simulink model "UZ_EnDat_be4_adding_bidirectional_clk_shift"  (R2024a)
settings: Solver=FixedStepDiscrete  StartTime=0  StopTime=0.02  FixedStep=1.0E-8  RelTol=1e-3
model workspace (MAT data in the model file):
  Select = 0
libraries: hdlsllib x776, simulink x28, simulink_extras x3
(part 6 of 9)

== system UZ_EnDat_be4_adding_bidirectional_clk_shift/UZ_ENDAT/timingprovideralternative/timingproviderold/Subsystem3 ==
  elapsed : Inport
  clkcnt : Inport  Port=2
  Compare To Constant1 : hdlsllib/Logic and Bit Operations/Compare To Constant  relop===  const=2  OutDataTypeStr=boolean
  Constant : Constant  Value=20  OutDataTypeStr=uint32  SampleTime=-1
  Delay1 : Delay  DelayLength=1
  Detect Increase : simulink/Logic and Bit Operations/Detect Increase  vinit=0  OutDataTypeStr=boolean
      settings: LibrarySourceBlock=|
      | hdlsllib/Logic and Bit
      | Operations/Detect
      | Increase
  Switch : Switch  Criteria=u2 > Threshold  SaturateOnIntegerOverflow=off  InputSameDT=off
  nsproduct : Product  OutDataTypeStr=uint32  RndMeth=Simplest  SaturateOnIntegerOverflow=on
  ns elapsed : Outport
  wires:
  Detect Increase/1 -> Switch/2
  clkcnt/1 -> Switch/1
  Switch/1 -> nsproduct/2, Delay1/1
  Delay1/1 -> Switch/3
  elapsed/1 -> Compare To Constant1/1
  nsproduct/1 -> ns elapsed/1  "ns elapsed"
  Constant/1 -> nsproduct/1
  Compare To Constant1/1 -> Detect Increase/1

== system UZ_EnDat_be4_adding_bidirectional_clk_shift/UZ_ENDAT/timingprovideralternative/timingproviderold/Subsystem4 ==
  reset : Inport
  Trigger : TriggerPort  VariantControl=(inherit)  PortDimensions=1
  Delay : Delay  Commented=through  DelayLength=1
  HDL Counter : hdlsllib/Sources/HDL Counter  CountType=Count limited  CountInit=0  CountStep=1  CountMax=214748364  CountFromType=Initial value  CountFrom=0  CountResetPort=on  CountLoadPort=off  CountEnbPort=off  CountDirPort=off  CountHitOutputPort=off  CountDataType=Unsigned  CountWordLen=32  CountFracLen=0  CountSampTime=1
  Scope : Scope
  valin1 : Outport  InitialOutput=0
  wires:
  reset/1 -> Delay/1
  HDL Counter/1 -> valin1/1, Scope/1
  Delay/1 -> HDL Counter/1

== system UZ_EnDat_be4_adding_bidirectional_clk_shift/UZ_ENDAT_ABZ_ADDON/ManualSerialize1/Storage1/prolonger ==
  in : Inport
  Delay4 : Delay  DelayLength=1
  Logical Operator5 : Logic  Operator=OR  AllPortsSameDT=off  OutDataTypeStr=boolean
  out : Outport
  wires:
  Logical Operator5/1 -> out/1
  in/1 -> Delay4/1, Logical Operator5/1
  Delay4/1 -> Logical Operator5/2

== system UZ_EnDat_be4_adding_bidirectional_clk_shift/UZ_ENDAT_ABZ_ADDON/ManualSerialize1/Storage2/prolonger ==
  in : Inport
  Delay4 : Delay  DelayLength=1
  Logical Operator5 : Logic  Operator=OR  Inputs=3  AllPortsSameDT=off  OutDataTypeStr=boolean
  out : Outport
  wires:
  Logical Operator5/1 -> out/1
  in/1 -> Logical Operator5/3, Delay4/1, Logical Operator5/1
  Delay4/1 -> Logical Operator5/2

== system UZ_EnDat_be4_adding_bidirectional_clk_shift/UZ_ENDAT_ABZ_ADDON/ManualSerialize1/nibblepadding6/padding ==
  in : Inport
  Bit Shift2 : hdlsllib/Logic and Bit Operations/Bit Shift  mode=Shift Right Logical  N=1
  Bit Slice2 : hdlsllib/Logic and Bit Operations/Bit Slice  lidx=0  ridx=0
  Data Type Conversion2 : DataTypeConversion  OutDataTypeStr=boolean  RndMeth=Nearest  SaturateOnIntegerOverflow=off
  Switch2 : Switch  Criteria=u2 > Threshold  SaturateOnIntegerOverflow=off  InputSameDT=off
  out : Outport
  wires:
  in/1 -> Bit Shift2/1, Switch2/1, Bit Slice2/1
  Bit Shift2/1 -> Switch2/3
  Data Type Conversion2/1 -> Switch2/2
  Bit Slice2/1 -> Data Type Conversion2/1
  Switch2/1 -> out/1

== system UZ_EnDat_be4_adding_bidirectional_clk_shift/UZ_ENDAT_ABZ_ADDON/ManualSerialize1/nibblepadding6/padding1 ==
  in : Inport
  Bit Shift2 : hdlsllib/Logic and Bit Operations/Bit Shift  mode=Shift Right Logical  N=1
  Bit Slice2 : hdlsllib/Logic and Bit Operations/Bit Slice  lidx=0  ridx=0
  Data Type Conversion2 : DataTypeConversion  OutDataTypeStr=boolean  RndMeth=Nearest  SaturateOnIntegerOverflow=off
  Switch2 : Switch  Criteria=u2 > Threshold  SaturateOnIntegerOverflow=off  InputSameDT=off
  out : Outport
  wires:
  in/1 -> Bit Shift2/1, Switch2/1, Bit Slice2/1
  Bit Shift2/1 -> Switch2/3
  Data Type Conversion2/1 -> Switch2/2
  Bit Slice2/1 -> Data Type Conversion2/1
  Switch2/1 -> out/1

== system UZ_EnDat_be4_adding_bidirectional_clk_shift/UZ_ENDAT_ABZ_ADDON/ManualSerialize1/nibblepadding6/padding2 ==
  in : Inport
  Bit Shift2 : hdlsllib/Logic and Bit Operations/Bit Shift  mode=Shift Right Logical  N=1
  Bit Slice2 : hdlsllib/Logic and Bit Operations/Bit Slice  lidx=0  ridx=0
  Data Type Conversion2 : DataTypeConversion  OutDataTypeStr=boolean  RndMeth=Nearest  SaturateOnIntegerOverflow=off
  Switch2 : Switch  Criteria=u2 > Threshold  SaturateOnIntegerOverflow=off  InputSameDT=off
  out : Outport
  wires:
  in/1 -> Bit Shift2/1, Switch2/1, Bit Slice2/1
  Bit Shift2/1 -> Switch2/3
  Data Type Conversion2/1 -> Switch2/2
  Bit Slice2/1 -> Data Type Conversion2/1
  Switch2/1 -> out/1

== system UZ_EnDat_be4_adding_bidirectional_clk_shift/UZ_ENDAT_ABZ_ADDON/ManualSerialize1/nibblepadding6/padding3 ==
  in : Inport
  Bit Shift2 : hdlsllib/Logic and Bit Operations/Bit Shift  mode=Shift Right Logical  N=1
  Bit Slice2 : hdlsllib/Logic and Bit Operations/Bit Slice  lidx=0  ridx=0
  Data Type Conversion2 : DataTypeConversion  OutDataTypeStr=boolean  RndMeth=Nearest  SaturateOnIntegerOverflow=off
  Switch2 : Switch  Criteria=u2 > Threshold  SaturateOnIntegerOverflow=off  InputSameDT=off
  out : Outport
  wires:
  in/1 -> Bit Shift2/1, Switch2/1, Bit Slice2/1
  Bit Shift2/1 -> Switch2/3
  Data Type Conversion2/1 -> Switch2/2
  Bit Slice2/1 -> Data Type Conversion2/1
  Switch2/1 -> out/1

== system UZ_EnDat_be4_adding_bidirectional_clk_shift/UZ_ENDAT_ABZ_ADDON/ManualSerialize1/padder/nibblepadding1 ==
  in : Inport
  padding : Subsystem  Commented=through
  padding1 : Subsystem
  padding2 : Subsystem
  padding3 : Subsystem
  out : Outport
  wires:
  in/1 -> padding3/1(in)
  padding2/1(out) -> padding1/1(in)
  padding3/1(out) -> padding2/1(in)
  padding1/1(out) -> padding/1(in)
  padding/1(out) -> out/1

== system UZ_EnDat_be4_adding_bidirectional_clk_shift/UZ_ENDAT_ABZ_ADDON/ManualSerialize1/padder/nibblepadding10 ==
  in : Inport
  padding : Subsystem  Commented=through
  padding1 : Subsystem
  padding2 : Subsystem
  padding3 : Subsystem
  out : Outport
  wires:
  in/1 -> padding3/1(in)
  padding2/1(out) -> padding1/1(in)
  padding3/1(out) -> padding2/1(in)
  padding1/1(out) -> padding/1(in)
  padding/1(out) -> out/1

== system UZ_EnDat_be4_adding_bidirectional_clk_shift/UZ_ENDAT_ABZ_ADDON/ManualSerialize1/padder/nibblepadding11 ==
  in : Inport
  padding : Subsystem  Commented=through
  padding1 : Subsystem
  padding2 : Subsystem
  padding3 : Subsystem
  out : Outport
  wires:
  in/1 -> padding3/1(in)
  padding2/1(out) -> padding1/1(in)
  padding3/1(out) -> padding2/1(in)
  padding1/1(out) -> padding/1(in)
  padding/1(out) -> out/1

== system UZ_EnDat_be4_adding_bidirectional_clk_shift/UZ_ENDAT_ABZ_ADDON/ManualSerialize1/padder/nibblepadding12 ==
  in : Inport
  padding : Subsystem  Commented=through
  padding1 : Subsystem
  padding2 : Subsystem
  padding3 : Subsystem
  out : Outport
  wires:
  in/1 -> padding3/1(in)
  padding2/1(out) -> padding1/1(in)
  padding3/1(out) -> padding2/1(in)
  padding1/1(out) -> padding/1(in)
  padding/1(out) -> out/1

== system UZ_EnDat_be4_adding_bidirectional_clk_shift/UZ_ENDAT_ABZ_ADDON/ManualSerialize1/padder/nibblepadding13 ==
  in : Inport
  padding : Subsystem  Commented=through
  padding1 : Subsystem
  padding2 : Subsystem
  padding3 : Subsystem
  out : Outport
  wires:
  in/1 -> padding3/1(in)
  padding2/1(out) -> padding1/1(in)
  padding3/1(out) -> padding2/1(in)
  padding1/1(out) -> padding/1(in)
  padding/1(out) -> out/1

== system UZ_EnDat_be4_adding_bidirectional_clk_shift/UZ_ENDAT_ABZ_ADDON/ManualSerialize1/padder/nibblepadding14 ==
  in : Inport
  padding : Subsystem  Commented=through
  padding1 : Subsystem
  padding2 : Subsystem
  padding3 : Subsystem
  out : Outport
  wires:
  in/1 -> padding3/1(in)
  padding2/1(out) -> padding1/1(in)
  padding3/1(out) -> padding2/1(in)
  padding1/1(out) -> padding/1(in)
  padding/1(out) -> out/1

== system UZ_EnDat_be4_adding_bidirectional_clk_shift/UZ_ENDAT_ABZ_ADDON/ManualSerialize1/padder/nibblepadding15 ==
  in : Inport
  padding : Subsystem  Commented=through
  padding1 : Subsystem
  padding2 : Subsystem
  padding3 : Subsystem
  out : Outport
  wires:
  in/1 -> padding3/1(in)
  padding2/1(out) -> padding1/1(in)
  padding3/1(out) -> padding2/1(in)
  padding1/1(out) -> padding/1(in)
  padding/1(out) -> out/1

== system UZ_EnDat_be4_adding_bidirectional_clk_shift/UZ_ENDAT_ABZ_ADDON/ManualSerialize1/padder/nibblepadding16 ==
  in : Inport
  padding : Subsystem  Commented=through
  padding1 : Subsystem
  padding2 : Subsystem
  padding3 : Subsystem
  out : Outport
  wires:
  in/1 -> padding3/1(in)
  padding2/1(out) -> padding1/1(in)
  padding3/1(out) -> padding2/1(in)
  padding1/1(out) -> padding/1(in)
  padding/1(out) -> out/1

== system UZ_EnDat_be4_adding_bidirectional_clk_shift/UZ_ENDAT_ABZ_ADDON/ManualSerialize1/padder/nibblepadding17 ==
  in : Inport
  padding : Subsystem  Commented=through
  padding1 : Subsystem
  padding2 : Subsystem
  padding3 : Subsystem
  out : Outport
  wires:
  in/1 -> padding3/1(in)
  padding2/1(out) -> padding1/1(in)
  padding3/1(out) -> padding2/1(in)
  padding1/1(out) -> padding/1(in)
  padding/1(out) -> out/1

== system UZ_EnDat_be4_adding_bidirectional_clk_shift/UZ_ENDAT_ABZ_ADDON/ManualSerialize1/padder/nibblepadding18 ==
  in : Inport
  padding : Subsystem  Commented=through
  padding1 : Subsystem
  padding2 : Subsystem
  padding3 : Subsystem
  out : Outport
  wires:
  in/1 -> padding3/1(in)
  padding2/1(out) -> padding1/1(in)
  padding3/1(out) -> padding2/1(in)
  padding1/1(out) -> padding/1(in)
  padding/1(out) -> out/1

== system UZ_EnDat_be4_adding_bidirectional_clk_shift/UZ_ENDAT_ABZ_ADDON/ManualSerialize1/padder/nibblepadding19 ==
  in : Inport
  padding : Subsystem  Commented=through
  padding1 : Subsystem
  padding2 : Subsystem
  padding3 : Subsystem
  out : Outport
  wires:
  in/1 -> padding3/1(in)
  padding2/1(out) -> padding1/1(in)
  padding3/1(out) -> padding2/1(in)
  padding1/1(out) -> padding/1(in)
  padding/1(out) -> out/1

== system UZ_EnDat_be4_adding_bidirectional_clk_shift/UZ_ENDAT_ABZ_ADDON/ManualSerialize1/padder/nibblepadding2 ==
  in : Inport
  padding : Subsystem  Commented=through
  padding1 : Subsystem
  padding2 : Subsystem
  padding3 : Subsystem
  out : Outport
  wires:
  in/1 -> padding3/1(in)
  padding2/1(out) -> padding1/1(in)
  padding3/1(out) -> padding2/1(in)
  padding1/1(out) -> padding/1(in)
  padding/1(out) -> out/1

== system UZ_EnDat_be4_adding_bidirectional_clk_shift/UZ_ENDAT_ABZ_ADDON/ManualSerialize1/padder/nibblepadding20 ==
  in : Inport
  padding : Subsystem  Commented=through
  padding1 : Subsystem
  padding2 : Subsystem
  padding3 : Subsystem
  out : Outport
  wires:
  in/1 -> padding3/1(in)
  padding2/1(out) -> padding1/1(in)
  padding3/1(out) -> padding2/1(in)
  padding1/1(out) -> padding/1(in)
  padding/1(out) -> out/1

== system UZ_EnDat_be4_adding_bidirectional_clk_shift/UZ_ENDAT_ABZ_ADDON/ManualSerialize1/padder/nibblepadding21 ==
  in : Inport
  padding : Subsystem  Commented=through
  padding1 : Subsystem
  padding2 : Subsystem
  padding3 : Subsystem
  out : Outport
  wires:
  in/1 -> padding3/1(in)
  padding2/1(out) -> padding1/1(in)
  padding3/1(out) -> padding2/1(in)
  padding1/1(out) -> padding/1(in)
  padding/1(out) -> out/1

== system UZ_EnDat_be4_adding_bidirectional_clk_shift/UZ_ENDAT_ABZ_ADDON/ManualSerialize1/padder/nibblepadding22 ==
  in : Inport
  padding : Subsystem  Commented=through
  padding1 : Subsystem
  padding2 : Subsystem
  padding3 : Subsystem
  out : Outport
  wires:
  in/1 -> padding3/1(in)
  padding2/1(out) -> padding1/1(in)
  padding3/1(out) -> padding2/1(in)
  padding1/1(out) -> padding/1(in)
  padding/1(out) -> out/1

== system UZ_EnDat_be4_adding_bidirectional_clk_shift/UZ_ENDAT_ABZ_ADDON/ManualSerialize1/padder/nibblepadding23 ==
  in : Inport
  padding : Subsystem  Commented=through
  padding1 : Subsystem
  padding2 : Subsystem
  padding3 : Subsystem
  out : Outport
  wires:
  in/1 -> padding3/1(in)
  padding2/1(out) -> padding1/1(in)
  padding3/1(out) -> padding2/1(in)
  padding1/1(out) -> padding/1(in)
  padding/1(out) -> out/1

== system UZ_EnDat_be4_adding_bidirectional_clk_shift/UZ_ENDAT_ABZ_ADDON/ManualSerialize1/padder/nibblepadding24 ==
  in : Inport
  padding : Subsystem  Commented=through
  padding1 : Subsystem
  padding2 : Subsystem
  padding3 : Subsystem
  out : Outport
  wires:
  in/1 -> padding3/1(in)
  padding2/1(out) -> padding1/1(in)
  padding3/1(out) -> padding2/1(in)
  padding1/1(out) -> padding/1(in)
  padding/1(out) -> out/1

== system UZ_EnDat_be4_adding_bidirectional_clk_shift/UZ_ENDAT_ABZ_ADDON/ManualSerialize1/padder/nibblepadding25 ==
  in : Inport
  padding : Subsystem  Commented=through
  padding1 : Subsystem
  padding2 : Subsystem
  padding3 : Subsystem
  out : Outport
  wires:
  in/1 -> padding3/1(in)
  padding2/1(out) -> padding1/1(in)
  padding3/1(out) -> padding2/1(in)
  padding1/1(out) -> padding/1(in)
  padding/1(out) -> out/1

== system UZ_EnDat_be4_adding_bidirectional_clk_shift/UZ_ENDAT_ABZ_ADDON/ManualSerialize1/padder/nibblepadding26 ==
  in : Inport
  padding : Subsystem  Commented=through
  padding1 : Subsystem
  padding2 : Subsystem
  padding3 : Subsystem
  out : Outport
  wires:
  in/1 -> padding3/1(in)
  padding2/1(out) -> padding1/1(in)
  padding3/1(out) -> padding2/1(in)
  padding1/1(out) -> padding/1(in)
  padding/1(out) -> out/1

== system UZ_EnDat_be4_adding_bidirectional_clk_shift/UZ_ENDAT_ABZ_ADDON/ManualSerialize1/padder/nibblepadding27 ==
  in : Inport
  padding : Subsystem  Commented=through
  padding1 : Subsystem
  padding2 : Subsystem
  padding3 : Subsystem
  out : Outport
  wires:
  in/1 -> padding3/1(in)
  padding2/1(out) -> padding1/1(in)
  padding3/1(out) -> padding2/1(in)
  padding1/1(out) -> padding/1(in)
  padding/1(out) -> out/1

== system UZ_EnDat_be4_adding_bidirectional_clk_shift/UZ_ENDAT_ABZ_ADDON/ManualSerialize1/padder/nibblepadding28 ==
  in : Inport
  padding : Subsystem  Commented=through
  padding1 : Subsystem
  padding2 : Subsystem
  padding3 : Subsystem
  out : Outport
  wires:
  in/1 -> padding3/1(in)
  padding2/1(out) -> padding1/1(in)
  padding3/1(out) -> padding2/1(in)
  padding1/1(out) -> padding/1(in)
  padding/1(out) -> out/1

== system UZ_EnDat_be4_adding_bidirectional_clk_shift/UZ_ENDAT_ABZ_ADDON/ManualSerialize1/padder/nibblepadding29 ==
  in : Inport
  padding : Subsystem  Commented=through
  padding1 : Subsystem
  padding2 : Subsystem
  padding3 : Subsystem
  out : Outport
  wires:
  in/1 -> padding3/1(in)
  padding2/1(out) -> padding1/1(in)
  padding3/1(out) -> padding2/1(in)
  padding1/1(out) -> padding/1(in)
  padding/1(out) -> out/1

== system UZ_EnDat_be4_adding_bidirectional_clk_shift/UZ_ENDAT_ABZ_ADDON/ManualSerialize1/padder/nibblepadding3 ==
  in : Inport
  padding : Subsystem  Commented=through
  padding1 : Subsystem
  padding2 : Subsystem
  padding3 : Subsystem
  out : Outport
  wires:
  in/1 -> padding3/1(in)
  padding2/1(out) -> padding1/1(in)
  padding3/1(out) -> padding2/1(in)
  padding1/1(out) -> padding/1(in)
  padding/1(out) -> out/1

== system UZ_EnDat_be4_adding_bidirectional_clk_shift/UZ_ENDAT_ABZ_ADDON/ManualSerialize1/padder/nibblepadding4 ==
  in : Inport
  padding : Subsystem  Commented=through
  padding1 : Subsystem
  padding2 : Subsystem
  padding3 : Subsystem
  out : Outport
  wires:
  in/1 -> padding3/1(in)
  padding2/1(out) -> padding1/1(in)
  padding3/1(out) -> padding2/1(in)
  padding1/1(out) -> padding/1(in)
  padding/1(out) -> out/1

== system UZ_EnDat_be4_adding_bidirectional_clk_shift/UZ_ENDAT_ABZ_ADDON/ManualSerialize1/padder/nibblepadding5 ==
  in : Inport
  padding : Subsystem  Commented=through
  padding1 : Subsystem
  padding2 : Subsystem
  padding3 : Subsystem
  out : Outport
  wires:
  in/1 -> padding3/1(in)
  padding2/1(out) -> padding1/1(in)
  padding3/1(out) -> padding2/1(in)
  padding1/1(out) -> padding/1(in)
  padding/1(out) -> out/1

== system UZ_EnDat_be4_adding_bidirectional_clk_shift/UZ_ENDAT_ABZ_ADDON/ManualSerialize1/padder/nibblepadding6 ==
  in : Inport
  padding : Subsystem  Commented=through
  padding1 : Subsystem
  padding2 : Subsystem
  padding3 : Subsystem
  out : Outport
  wires:
  in/1 -> padding3/1(in)
  padding2/1(out) -> padding1/1(in)
  padding3/1(out) -> padding2/1(in)
  padding1/1(out) -> padding/1(in)
  padding/1(out) -> out/1

== system UZ_EnDat_be4_adding_bidirectional_clk_shift/UZ_ENDAT_ABZ_ADDON/ManualSerialize1/padder/nibblepadding7 ==
  in : Inport
  padding : Subsystem  Commented=through
  padding1 : Subsystem
  padding2 : Subsystem
  padding3 : Subsystem
  out : Outport
  wires:
  in/1 -> padding3/1(in)
  padding2/1(out) -> padding1/1(in)
  padding3/1(out) -> padding2/1(in)
  padding1/1(out) -> padding/1(in)
  padding/1(out) -> out/1

== system UZ_EnDat_be4_adding_bidirectional_clk_shift/UZ_ENDAT_ABZ_ADDON/ManualSerialize1/padder/nibblepadding8 ==
  in : Inport
  padding : Subsystem  Commented=through
  padding1 : Subsystem
  padding2 : Subsystem
  padding3 : Subsystem
  out : Outport
  wires:
  in/1 -> padding3/1(in)
  padding2/1(out) -> padding1/1(in)
  padding3/1(out) -> padding2/1(in)
  padding1/1(out) -> padding/1(in)
  padding/1(out) -> out/1

== system UZ_EnDat_be4_adding_bidirectional_clk_shift/UZ_ENDAT_ABZ_ADDON/ManualSerialize1/padder/nibblepadding9 ==
  in : Inport
  padding : Subsystem  Commented=through
  padding1 : Subsystem
  padding2 : Subsystem
  padding3 : Subsystem
  out : Outport
  wires:
  in/1 -> padding3/1(in)
  padding2/1(out) -> padding1/1(in)
  padding3/1(out) -> padding2/1(in)
  padding1/1(out) -> padding/1(in)
  padding/1(out) -> out/1

== system UZ_EnDat_be4_adding_bidirectional_clk_shift/UZ_ENDAT_ABZ_ADDON/responseslicer5/ENDAT23BITREVERSER/32BITREVERSE ==
  in : Inport
  16BITREVERSER : Subsystem
  16BITREVERSER1 : Subsystem
  Bit Concat : hdlsllib/Logic and Bit Operations/Bit Concat  numInputs=2
  Bit Slice : hdlsllib/Logic and Bit Operations/Bit Slice  lidx=15  ridx=0
  Bit Slice1 : hdlsllib/Logic and Bit Operations/Bit Slice  lidx=31  ridx=16
  out : Outport
  wires:
  in/1 -> Bit Slice1/1, Bit Slice/1
  16BITREVERSER/1(out) -> Bit Concat/1
  16BITREVERSER1/1(out) -> Bit Concat/2
  Bit Concat/1 -> out/1
  Bit Slice/1 -> 16BITREVERSER/1(in)
  Bit Slice1/1 -> 16BITREVERSER1/1(in)

== system UZ_EnDat_be4_adding_bidirectional_clk_shift/UZ_ENDAT/ManualDeserialize/padder/nibblepadding1/padding ==
  in : Inport
  Bit Shift2 : hdlsllib/Logic and Bit Operations/Bit Shift  mode=Shift Right Logical  N=1
  Bit Slice2 : hdlsllib/Logic and Bit Operations/Bit Slice  lidx=0  ridx=0
  Data Type Conversion2 : DataTypeConversion  OutDataTypeStr=boolean  RndMeth=Nearest  SaturateOnIntegerOverflow=off
  Switch2 : Switch  Criteria=u2 > Threshold  SaturateOnIntegerOverflow=off  InputSameDT=off
  out : Outport
  wires:
  in/1 -> Bit Shift2/1, Switch2/1, Bit Slice2/1
  Bit Shift2/1 -> Switch2/3
  Data Type Conversion2/1 -> Switch2/2
  Bit Slice2/1 -> Data Type Conversion2/1
  Switch2/1 -> out/1

== system UZ_EnDat_be4_adding_bidirectional_clk_shift/UZ_ENDAT/ManualDeserialize/padder/nibblepadding1/padding1 ==
  in : Inport
  Bit Shift2 : hdlsllib/Logic and Bit Operations/Bit Shift  mode=Shift Right Logical  N=1
  Bit Slice2 : hdlsllib/Logic and Bit Operations/Bit Slice  lidx=0  ridx=0
  Data Type Conversion2 : DataTypeConversion  OutDataTypeStr=boolean  RndMeth=Nearest  SaturateOnIntegerOverflow=off
  Switch2 : Switch  Criteria=u2 > Threshold  SaturateOnIntegerOverflow=off  InputSameDT=off
  out : Outport
  wires:
  in/1 -> Bit Shift2/1, Switch2/1, Bit Slice2/1
  Bit Shift2/1 -> Switch2/3
  Data Type Conversion2/1 -> Switch2/2
  Bit Slice2/1 -> Data Type Conversion2/1
  Switch2/1 -> out/1

== system UZ_EnDat_be4_adding_bidirectional_clk_shift/UZ_ENDAT/ManualDeserialize/padder/nibblepadding1/padding2 ==
  in : Inport
  Bit Shift2 : hdlsllib/Logic and Bit Operations/Bit Shift  mode=Shift Right Logical  N=1
  Bit Slice2 : hdlsllib/Logic and Bit Operations/Bit Slice  lidx=0  ridx=0
  Data Type Conversion2 : DataTypeConversion  OutDataTypeStr=boolean  RndMeth=Nearest  SaturateOnIntegerOverflow=off
  Switch2 : Switch  Criteria=u2 > Threshold  SaturateOnIntegerOverflow=off  InputSameDT=off
  out : Outport
  wires:
  in/1 -> Bit Shift2/1, Switch2/1, Bit Slice2/1
  Bit Shift2/1 -> Switch2/3
  Data Type Conversion2/1 -> Switch2/2
  Bit Slice2/1 -> Data Type Conversion2/1
  Switch2/1 -> out/1

== system UZ_EnDat_be4_adding_bidirectional_clk_shift/UZ_ENDAT/ManualDeserialize/padder/nibblepadding1/padding3 ==
  in : Inport
  Bit Shift2 : hdlsllib/Logic and Bit Operations/Bit Shift  mode=Shift Right Logical  N=1
  Bit Slice2 : hdlsllib/Logic and Bit Operations/Bit Slice  lidx=0  ridx=0
  Data Type Conversion2 : DataTypeConversion  OutDataTypeStr=boolean  RndMeth=Nearest  SaturateOnIntegerOverflow=off
  Switch2 : Switch  Criteria=u2 > Threshold  SaturateOnIntegerOverflow=off  InputSameDT=off
  out : Outport
  wires:
  in/1 -> Bit Shift2/1, Switch2/1, Bit Slice2/1
  Bit Shift2/1 -> Switch2/3
  Data Type Conversion2/1 -> Switch2/2
  Bit Slice2/1 -> Data Type Conversion2/1
  Switch2/1 -> out/1

== system UZ_EnDat_be4_adding_bidirectional_clk_shift/UZ_ENDAT/ManualDeserialize/padder/nibblepadding10/padding ==
  in : Inport
  Bit Shift2 : hdlsllib/Logic and Bit Operations/Bit Shift  mode=Shift Right Logical  N=1
  Bit Slice2 : hdlsllib/Logic and Bit Operations/Bit Slice  lidx=0  ridx=0
  Data Type Conversion2 : DataTypeConversion  OutDataTypeStr=boolean  RndMeth=Nearest  SaturateOnIntegerOverflow=off
  Switch2 : Switch  Criteria=u2 > Threshold  SaturateOnIntegerOverflow=off  InputSameDT=off
  out : Outport
  wires:
  in/1 -> Bit Shift2/1, Switch2/1, Bit Slice2/1
  Bit Shift2/1 -> Switch2/3
  Data Type Conversion2/1 -> Switch2/2
  Bit Slice2/1 -> Data Type Conversion2/1
  Switch2/1 -> out/1

== system UZ_EnDat_be4_adding_bidirectional_clk_shift/UZ_ENDAT/ManualDeserialize/padder/nibblepadding10/padding1 ==
  in : Inport
  Bit Shift2 : hdlsllib/Logic and Bit Operations/Bit Shift  mode=Shift Right Logical  N=1
  Bit Slice2 : hdlsllib/Logic and Bit Operations/Bit Slice  lidx=0  ridx=0
  Data Type Conversion2 : DataTypeConversion  OutDataTypeStr=boolean  RndMeth=Nearest  SaturateOnIntegerOverflow=off
  Switch2 : Switch  Criteria=u2 > Threshold  SaturateOnIntegerOverflow=off  InputSameDT=off
  out : Outport
  wires:
  in/1 -> Bit Shift2/1, Switch2/1, Bit Slice2/1
  Bit Shift2/1 -> Switch2/3
  Data Type Conversion2/1 -> Switch2/2
  Bit Slice2/1 -> Data Type Conversion2/1
  Switch2/1 -> out/1

== system UZ_EnDat_be4_adding_bidirectional_clk_shift/UZ_ENDAT/ManualDeserialize/padder/nibblepadding10/padding2 ==
  in : Inport
  Bit Shift2 : hdlsllib/Logic and Bit Operations/Bit Shift  mode=Shift Right Logical  N=1
  Bit Slice2 : hdlsllib/Logic and Bit Operations/Bit Slice  lidx=0  ridx=0
  Data Type Conversion2 : DataTypeConversion  OutDataTypeStr=boolean  RndMeth=Nearest  SaturateOnIntegerOverflow=off
  Switch2 : Switch  Criteria=u2 > Threshold  SaturateOnIntegerOverflow=off  InputSameDT=off
  out : Outport
  wires:
  in/1 -> Bit Shift2/1, Switch2/1, Bit Slice2/1
  Bit Shift2/1 -> Switch2/3
  Data Type Conversion2/1 -> Switch2/2
  Bit Slice2/1 -> Data Type Conversion2/1
  Switch2/1 -> out/1

== system UZ_EnDat_be4_adding_bidirectional_clk_shift/UZ_ENDAT/ManualDeserialize/padder/nibblepadding10/padding3 ==
  in : Inport
  Bit Shift2 : hdlsllib/Logic and Bit Operations/Bit Shift  mode=Shift Right Logical  N=1
  Bit Slice2 : hdlsllib/Logic and Bit Operations/Bit Slice  lidx=0  ridx=0
  Data Type Conversion2 : DataTypeConversion  OutDataTypeStr=boolean  RndMeth=Nearest  SaturateOnIntegerOverflow=off
  Switch2 : Switch  Criteria=u2 > Threshold  SaturateOnIntegerOverflow=off  InputSameDT=off
  out : Outport
  wires:
  in/1 -> Bit Shift2/1, Switch2/1, Bit Slice2/1
  Bit Shift2/1 -> Switch2/3
  Data Type Conversion2/1 -> Switch2/2
  Bit Slice2/1 -> Data Type Conversion2/1
  Switch2/1 -> out/1

== system UZ_EnDat_be4_adding_bidirectional_clk_shift/UZ_ENDAT/ManualDeserialize/padder/nibblepadding11/padding ==
  in : Inport
  Bit Shift2 : hdlsllib/Logic and Bit Operations/Bit Shift  mode=Shift Right Logical  N=1
  Bit Slice2 : hdlsllib/Logic and Bit Operations/Bit Slice  lidx=0  ridx=0
  Data Type Conversion2 : DataTypeConversion  OutDataTypeStr=boolean  RndMeth=Nearest  SaturateOnIntegerOverflow=off
  Switch2 : Switch  Criteria=u2 > Threshold  SaturateOnIntegerOverflow=off  InputSameDT=off
  out : Outport
  wires:
  in/1 -> Bit Shift2/1, Switch2/1, Bit Slice2/1
  Bit Shift2/1 -> Switch2/3
  Data Type Conversion2/1 -> Switch2/2
  Bit Slice2/1 -> Data Type Conversion2/1
  Switch2/1 -> out/1

== system UZ_EnDat_be4_adding_bidirectional_clk_shift/UZ_ENDAT/ManualDeserialize/padder/nibblepadding11/padding1 ==
  in : Inport
  Bit Shift2 : hdlsllib/Logic and Bit Operations/Bit Shift  mode=Shift Right Logical  N=1
  Bit Slice2 : hdlsllib/Logic and Bit Operations/Bit Slice  lidx=0  ridx=0
  Data Type Conversion2 : DataTypeConversion  OutDataTypeStr=boolean  RndMeth=Nearest  SaturateOnIntegerOverflow=off
  Switch2 : Switch  Criteria=u2 > Threshold  SaturateOnIntegerOverflow=off  InputSameDT=off
  out : Outport
  wires:
  in/1 -> Bit Shift2/1, Switch2/1, Bit Slice2/1
  Bit Shift2/1 -> Switch2/3
  Data Type Conversion2/1 -> Switch2/2
  Bit Slice2/1 -> Data Type Conversion2/1
  Switch2/1 -> out/1

== system UZ_EnDat_be4_adding_bidirectional_clk_shift/UZ_ENDAT/ManualDeserialize/padder/nibblepadding11/padding2 ==
  in : Inport
  Bit Shift2 : hdlsllib/Logic and Bit Operations/Bit Shift  mode=Shift Right Logical  N=1
  Bit Slice2 : hdlsllib/Logic and Bit Operations/Bit Slice  lidx=0  ridx=0
  Data Type Conversion2 : DataTypeConversion  OutDataTypeStr=boolean  RndMeth=Nearest  SaturateOnIntegerOverflow=off
  Switch2 : Switch  Criteria=u2 > Threshold  SaturateOnIntegerOverflow=off  InputSameDT=off
  out : Outport
  wires:
  in/1 -> Bit Shift2/1, Switch2/1, Bit Slice2/1
  Bit Shift2/1 -> Switch2/3
  Data Type Conversion2/1 -> Switch2/2
  Bit Slice2/1 -> Data Type Conversion2/1
  Switch2/1 -> out/1

== system UZ_EnDat_be4_adding_bidirectional_clk_shift/UZ_ENDAT/ManualDeserialize/padder/nibblepadding11/padding3 ==
  in : Inport
  Bit Shift2 : hdlsllib/Logic and Bit Operations/Bit Shift  mode=Shift Right Logical  N=1
  Bit Slice2 : hdlsllib/Logic and Bit Operations/Bit Slice  lidx=0  ridx=0
  Data Type Conversion2 : DataTypeConversion  OutDataTypeStr=boolean  RndMeth=Nearest  SaturateOnIntegerOverflow=off
  Switch2 : Switch  Criteria=u2 > Threshold  SaturateOnIntegerOverflow=off  InputSameDT=off
  out : Outport
  wires:
  in/1 -> Bit Shift2/1, Switch2/1, Bit Slice2/1
  Bit Shift2/1 -> Switch2/3
  Data Type Conversion2/1 -> Switch2/2
  Bit Slice2/1 -> Data Type Conversion2/1
  Switch2/1 -> out/1

== system UZ_EnDat_be4_adding_bidirectional_clk_shift/UZ_ENDAT/ManualDeserialize/padder/nibblepadding12/padding ==
  in : Inport
  Bit Shift2 : hdlsllib/Logic and Bit Operations/Bit Shift  mode=Shift Right Logical  N=1
  Bit Slice2 : hdlsllib/Logic and Bit Operations/Bit Slice  lidx=0  ridx=0
  Data Type Conversion2 : DataTypeConversion  OutDataTypeStr=boolean  RndMeth=Nearest  SaturateOnIntegerOverflow=off
  Switch2 : Switch  Criteria=u2 > Threshold  SaturateOnIntegerOverflow=off  InputSameDT=off
  out : Outport
  wires:
  in/1 -> Bit Shift2/1, Switch2/1, Bit Slice2/1
  Bit Shift2/1 -> Switch2/3
  Data Type Conversion2/1 -> Switch2/2
  Bit Slice2/1 -> Data Type Conversion2/1
  Switch2/1 -> out/1

== system UZ_EnDat_be4_adding_bidirectional_clk_shift/UZ_ENDAT/ManualDeserialize/padder/nibblepadding12/padding1 ==
  in : Inport
  Bit Shift2 : hdlsllib/Logic and Bit Operations/Bit Shift  mode=Shift Right Logical  N=1
  Bit Slice2 : hdlsllib/Logic and Bit Operations/Bit Slice  lidx=0  ridx=0
  Data Type Conversion2 : DataTypeConversion  OutDataTypeStr=boolean  RndMeth=Nearest  SaturateOnIntegerOverflow=off
  Switch2 : Switch  Criteria=u2 > Threshold  SaturateOnIntegerOverflow=off  InputSameDT=off
  out : Outport
  wires:
  in/1 -> Bit Shift2/1, Switch2/1, Bit Slice2/1
  Bit Shift2/1 -> Switch2/3
  Data Type Conversion2/1 -> Switch2/2
  Bit Slice2/1 -> Data Type Conversion2/1
  Switch2/1 -> out/1

== system UZ_EnDat_be4_adding_bidirectional_clk_shift/UZ_ENDAT/ManualDeserialize/padder/nibblepadding12/padding2 ==
  in : Inport
  Bit Shift2 : hdlsllib/Logic and Bit Operations/Bit Shift  mode=Shift Right Logical  N=1
  Bit Slice2 : hdlsllib/Logic and Bit Operations/Bit Slice  lidx=0  ridx=0
  Data Type Conversion2 : DataTypeConversion  OutDataTypeStr=boolean  RndMeth=Nearest  SaturateOnIntegerOverflow=off
  Switch2 : Switch  Criteria=u2 > Threshold  SaturateOnIntegerOverflow=off  InputSameDT=off
  out : Outport
  wires:
  in/1 -> Bit Shift2/1, Switch2/1, Bit Slice2/1
  Bit Shift2/1 -> Switch2/3
  Data Type Conversion2/1 -> Switch2/2
  Bit Slice2/1 -> Data Type Conversion2/1
  Switch2/1 -> out/1

== system UZ_EnDat_be4_adding_bidirectional_clk_shift/UZ_ENDAT/ManualDeserialize/padder/nibblepadding12/padding3 ==
  in : Inport
  Bit Shift2 : hdlsllib/Logic and Bit Operations/Bit Shift  mode=Shift Right Logical  N=1
  Bit Slice2 : hdlsllib/Logic and Bit Operations/Bit Slice  lidx=0  ridx=0
  Data Type Conversion2 : DataTypeConversion  OutDataTypeStr=boolean  RndMeth=Nearest  SaturateOnIntegerOverflow=off
  Switch2 : Switch  Criteria=u2 > Threshold  SaturateOnIntegerOverflow=off  InputSameDT=off
  out : Outport
  wires:
  in/1 -> Bit Shift2/1, Switch2/1, Bit Slice2/1
  Bit Shift2/1 -> Switch2/3
  Data Type Conversion2/1 -> Switch2/2
  Bit Slice2/1 -> Data Type Conversion2/1
  Switch2/1 -> out/1

== system UZ_EnDat_be4_adding_bidirectional_clk_shift/UZ_ENDAT/ManualDeserialize/padder/nibblepadding13/padding ==
  in : Inport
  Bit Shift2 : hdlsllib/Logic and Bit Operations/Bit Shift  mode=Shift Right Logical  N=1
  Bit Slice2 : hdlsllib/Logic and Bit Operations/Bit Slice  lidx=0  ridx=0
  Data Type Conversion2 : DataTypeConversion  OutDataTypeStr=boolean  RndMeth=Nearest  SaturateOnIntegerOverflow=off
  Switch2 : Switch  Criteria=u2 > Threshold  SaturateOnIntegerOverflow=off  InputSameDT=off
  out : Outport
  wires:
  in/1 -> Bit Shift2/1, Switch2/1, Bit Slice2/1
  Bit Shift2/1 -> Switch2/3
  Data Type Conversion2/1 -> Switch2/2
  Bit Slice2/1 -> Data Type Conversion2/1
  Switch2/1 -> out/1

== system UZ_EnDat_be4_adding_bidirectional_clk_shift/UZ_ENDAT/ManualDeserialize/padder/nibblepadding13/padding1 ==
  in : Inport
  Bit Shift2 : hdlsllib/Logic and Bit Operations/Bit Shift  mode=Shift Right Logical  N=1
  Bit Slice2 : hdlsllib/Logic and Bit Operations/Bit Slice  lidx=0  ridx=0
  Data Type Conversion2 : DataTypeConversion  OutDataTypeStr=boolean  RndMeth=Nearest  SaturateOnIntegerOverflow=off
  Switch2 : Switch  Criteria=u2 > Threshold  SaturateOnIntegerOverflow=off  InputSameDT=off
  out : Outport
  wires:
  in/1 -> Bit Shift2/1, Switch2/1, Bit Slice2/1
  Bit Shift2/1 -> Switch2/3
  Data Type Conversion2/1 -> Switch2/2
  Bit Slice2/1 -> Data Type Conversion2/1
  Switch2/1 -> out/1

== system UZ_EnDat_be4_adding_bidirectional_clk_shift/UZ_ENDAT/ManualDeserialize/padder/nibblepadding13/padding2 ==
  in : Inport
  Bit Shift2 : hdlsllib/Logic and Bit Operations/Bit Shift  mode=Shift Right Logical  N=1
  Bit Slice2 : hdlsllib/Logic and Bit Operations/Bit Slice  lidx=0  ridx=0
  Data Type Conversion2 : DataTypeConversion  OutDataTypeStr=boolean  RndMeth=Nearest  SaturateOnIntegerOverflow=off
  Switch2 : Switch  Criteria=u2 > Threshold  SaturateOnIntegerOverflow=off  InputSameDT=off
  out : Outport
  wires:
  in/1 -> Bit Shift2/1, Switch2/1, Bit Slice2/1
  Bit Shift2/1 -> Switch2/3
  Data Type Conversion2/1 -> Switch2/2
  Bit Slice2/1 -> Data Type Conversion2/1
  Switch2/1 -> out/1

== system UZ_EnDat_be4_adding_bidirectional_clk_shift/UZ_ENDAT/ManualDeserialize/padder/nibblepadding13/padding3 ==
  in : Inport
  Bit Shift2 : hdlsllib/Logic and Bit Operations/Bit Shift  mode=Shift Right Logical  N=1
  Bit Slice2 : hdlsllib/Logic and Bit Operations/Bit Slice  lidx=0  ridx=0
  Data Type Conversion2 : DataTypeConversion  OutDataTypeStr=boolean  RndMeth=Nearest  SaturateOnIntegerOverflow=off
  Switch2 : Switch  Criteria=u2 > Threshold  SaturateOnIntegerOverflow=off  InputSameDT=off
  out : Outport
  wires:
  in/1 -> Bit Shift2/1, Switch2/1, Bit Slice2/1
  Bit Shift2/1 -> Switch2/3
  Data Type Conversion2/1 -> Switch2/2
  Bit Slice2/1 -> Data Type Conversion2/1
  Switch2/1 -> out/1

== system UZ_EnDat_be4_adding_bidirectional_clk_shift/UZ_ENDAT/ManualDeserialize/padder/nibblepadding14/padding ==
  in : Inport
  Bit Shift2 : hdlsllib/Logic and Bit Operations/Bit Shift  mode=Shift Right Logical  N=1
  Bit Slice2 : hdlsllib/Logic and Bit Operations/Bit Slice  lidx=0  ridx=0
  Data Type Conversion2 : DataTypeConversion  OutDataTypeStr=boolean  RndMeth=Nearest  SaturateOnIntegerOverflow=off
  Switch2 : Switch  Criteria=u2 > Threshold  SaturateOnIntegerOverflow=off  InputSameDT=off
  out : Outport
  wires:
  in/1 -> Bit Shift2/1, Switch2/1, Bit Slice2/1
  Bit Shift2/1 -> Switch2/3
  Data Type Conversion2/1 -> Switch2/2
  Bit Slice2/1 -> Data Type Conversion2/1
  Switch2/1 -> out/1

== system UZ_EnDat_be4_adding_bidirectional_clk_shift/UZ_ENDAT/ManualDeserialize/padder/nibblepadding14/padding1 ==
  in : Inport
  Bit Shift2 : hdlsllib/Logic and Bit Operations/Bit Shift  mode=Shift Right Logical  N=1
  Bit Slice2 : hdlsllib/Logic and Bit Operations/Bit Slice  lidx=0  ridx=0
  Data Type Conversion2 : DataTypeConversion  OutDataTypeStr=boolean  RndMeth=Nearest  SaturateOnIntegerOverflow=off
  Switch2 : Switch  Criteria=u2 > Threshold  SaturateOnIntegerOverflow=off  InputSameDT=off
  out : Outport
  wires:
  in/1 -> Bit Shift2/1, Switch2/1, Bit Slice2/1
  Bit Shift2/1 -> Switch2/3
  Data Type Conversion2/1 -> Switch2/2
  Bit Slice2/1 -> Data Type Conversion2/1
  Switch2/1 -> out/1

== system UZ_EnDat_be4_adding_bidirectional_clk_shift/UZ_ENDAT/ManualDeserialize/padder/nibblepadding14/padding2 ==
  in : Inport
  Bit Shift2 : hdlsllib/Logic and Bit Operations/Bit Shift  mode=Shift Right Logical  N=1
  Bit Slice2 : hdlsllib/Logic and Bit Operations/Bit Slice  lidx=0  ridx=0
  Data Type Conversion2 : DataTypeConversion  OutDataTypeStr=boolean  RndMeth=Nearest  SaturateOnIntegerOverflow=off
  Switch2 : Switch  Criteria=u2 > Threshold  SaturateOnIntegerOverflow=off  InputSameDT=off
  out : Outport
  wires:
  in/1 -> Bit Shift2/1, Switch2/1, Bit Slice2/1
  Bit Shift2/1 -> Switch2/3
  Data Type Conversion2/1 -> Switch2/2
  Bit Slice2/1 -> Data Type Conversion2/1
  Switch2/1 -> out/1

== system UZ_EnDat_be4_adding_bidirectional_clk_shift/UZ_ENDAT/ManualDeserialize/padder/nibblepadding14/padding3 ==
  in : Inport
  Bit Shift2 : hdlsllib/Logic and Bit Operations/Bit Shift  mode=Shift Right Logical  N=1
  Bit Slice2 : hdlsllib/Logic and Bit Operations/Bit Slice  lidx=0  ridx=0
  Data Type Conversion2 : DataTypeConversion  OutDataTypeStr=boolean  RndMeth=Nearest  SaturateOnIntegerOverflow=off
  Switch2 : Switch  Criteria=u2 > Threshold  SaturateOnIntegerOverflow=off  InputSameDT=off
  out : Outport
  wires:
  in/1 -> Bit Shift2/1, Switch2/1, Bit Slice2/1
  Bit Shift2/1 -> Switch2/3
  Data Type Conversion2/1 -> Switch2/2
  Bit Slice2/1 -> Data Type Conversion2/1
  Switch2/1 -> out/1

== system UZ_EnDat_be4_adding_bidirectional_clk_shift/UZ_ENDAT/ManualDeserialize/padder/nibblepadding15/padding ==
  in : Inport
  Bit Shift2 : hdlsllib/Logic and Bit Operations/Bit Shift  mode=Shift Right Logical  N=1
  Bit Slice2 : hdlsllib/Logic and Bit Operations/Bit Slice  lidx=0  ridx=0
  Data Type Conversion2 : DataTypeConversion  OutDataTypeStr=boolean  RndMeth=Nearest  SaturateOnIntegerOverflow=off
  Switch2 : Switch  Criteria=u2 > Threshold  SaturateOnIntegerOverflow=off  InputSameDT=off
  out : Outport
  wires:
  in/1 -> Bit Shift2/1, Switch2/1, Bit Slice2/1
  Bit Shift2/1 -> Switch2/3
  Data Type Conversion2/1 -> Switch2/2
  Bit Slice2/1 -> Data Type Conversion2/1
  Switch2/1 -> out/1

== system UZ_EnDat_be4_adding_bidirectional_clk_shift/UZ_ENDAT/ManualDeserialize/padder/nibblepadding15/padding1 ==
  in : Inport
  Bit Shift2 : hdlsllib/Logic and Bit Operations/Bit Shift  mode=Shift Right Logical  N=1
  Bit Slice2 : hdlsllib/Logic and Bit Operations/Bit Slice  lidx=0  ridx=0
  Data Type Conversion2 : DataTypeConversion  OutDataTypeStr=boolean  RndMeth=Nearest  SaturateOnIntegerOverflow=off
  Switch2 : Switch  Criteria=u2 > Threshold  SaturateOnIntegerOverflow=off  InputSameDT=off
  out : Outport
  wires:
  in/1 -> Bit Shift2/1, Switch2/1, Bit Slice2/1
  Bit Shift2/1 -> Switch2/3
  Data Type Conversion2/1 -> Switch2/2
  Bit Slice2/1 -> Data Type Conversion2/1
  Switch2/1 -> out/1

== system UZ_EnDat_be4_adding_bidirectional_clk_shift/UZ_ENDAT/ManualDeserialize/padder/nibblepadding15/padding2 ==
  in : Inport
  Bit Shift2 : hdlsllib/Logic and Bit Operations/Bit Shift  mode=Shift Right Logical  N=1
  Bit Slice2 : hdlsllib/Logic and Bit Operations/Bit Slice  lidx=0  ridx=0
  Data Type Conversion2 : DataTypeConversion  OutDataTypeStr=boolean  RndMeth=Nearest  SaturateOnIntegerOverflow=off
  Switch2 : Switch  Criteria=u2 > Threshold  SaturateOnIntegerOverflow=off  InputSameDT=off
  out : Outport
  wires:
  in/1 -> Bit Shift2/1, Switch2/1, Bit Slice2/1
  Bit Shift2/1 -> Switch2/3
  Data Type Conversion2/1 -> Switch2/2
  Bit Slice2/1 -> Data Type Conversion2/1
  Switch2/1 -> out/1

== system UZ_EnDat_be4_adding_bidirectional_clk_shift/UZ_ENDAT/ManualDeserialize/padder/nibblepadding15/padding3 ==
  in : Inport
  Bit Shift2 : hdlsllib/Logic and Bit Operations/Bit Shift  mode=Shift Right Logical  N=1
  Bit Slice2 : hdlsllib/Logic and Bit Operations/Bit Slice  lidx=0  ridx=0
  Data Type Conversion2 : DataTypeConversion  OutDataTypeStr=boolean  RndMeth=Nearest  SaturateOnIntegerOverflow=off
  Switch2 : Switch  Criteria=u2 > Threshold  SaturateOnIntegerOverflow=off  InputSameDT=off
  out : Outport
  wires:
  in/1 -> Bit Shift2/1, Switch2/1, Bit Slice2/1
  Bit Shift2/1 -> Switch2/3
  Data Type Conversion2/1 -> Switch2/2
  Bit Slice2/1 -> Data Type Conversion2/1
  Switch2/1 -> out/1

== system UZ_EnDat_be4_adding_bidirectional_clk_shift/UZ_ENDAT/ManualDeserialize/padder/nibblepadding16/padding ==
  in : Inport
  Bit Shift2 : hdlsllib/Logic and Bit Operations/Bit Shift  mode=Shift Right Logical  N=1
  Bit Slice2 : hdlsllib/Logic and Bit Operations/Bit Slice  lidx=0  ridx=0
  Data Type Conversion2 : DataTypeConversion  OutDataTypeStr=boolean  RndMeth=Nearest  SaturateOnIntegerOverflow=off
  Switch2 : Switch  Criteria=u2 > Threshold  SaturateOnIntegerOverflow=off  InputSameDT=off
  out : Outport
  wires:
  in/1 -> Bit Shift2/1, Switch2/1, Bit Slice2/1
  Bit Shift2/1 -> Switch2/3
  Data Type Conversion2/1 -> Switch2/2
  Bit Slice2/1 -> Data Type Conversion2/1
  Switch2/1 -> out/1

== system UZ_EnDat_be4_adding_bidirectional_clk_shift/UZ_ENDAT/ManualDeserialize/padder/nibblepadding16/padding1 ==
  in : Inport
  Bit Shift2 : hdlsllib/Logic and Bit Operations/Bit Shift  mode=Shift Right Logical  N=1
  Bit Slice2 : hdlsllib/Logic and Bit Operations/Bit Slice  lidx=0  ridx=0
  Data Type Conversion2 : DataTypeConversion  OutDataTypeStr=boolean  RndMeth=Nearest  SaturateOnIntegerOverflow=off
  Switch2 : Switch  Criteria=u2 > Threshold  SaturateOnIntegerOverflow=off  InputSameDT=off
  out : Outport
  wires:
  in/1 -> Bit Shift2/1, Switch2/1, Bit Slice2/1
  Bit Shift2/1 -> Switch2/3
  Data Type Conversion2/1 -> Switch2/2
  Bit Slice2/1 -> Data Type Conversion2/1
  Switch2/1 -> out/1

== system UZ_EnDat_be4_adding_bidirectional_clk_shift/UZ_ENDAT/ManualDeserialize/padder/nibblepadding16/padding2 ==
  in : Inport
  Bit Shift2 : hdlsllib/Logic and Bit Operations/Bit Shift  mode=Shift Right Logical  N=1
  Bit Slice2 : hdlsllib/Logic and Bit Operations/Bit Slice  lidx=0  ridx=0
  Data Type Conversion2 : DataTypeConversion  OutDataTypeStr=boolean  RndMeth=Nearest  SaturateOnIntegerOverflow=off
  Switch2 : Switch  Criteria=u2 > Threshold  SaturateOnIntegerOverflow=off  InputSameDT=off
  out : Outport
  wires:
  in/1 -> Bit Shift2/1, Switch2/1, Bit Slice2/1
  Bit Shift2/1 -> Switch2/3
  Data Type Conversion2/1 -> Switch2/2
  Bit Slice2/1 -> Data Type Conversion2/1
  Switch2/1 -> out/1

== system UZ_EnDat_be4_adding_bidirectional_clk_shift/UZ_ENDAT/ManualDeserialize/padder/nibblepadding16/padding3 ==
  in : Inport
  Bit Shift2 : hdlsllib/Logic and Bit Operations/Bit Shift  mode=Shift Right Logical  N=1
  Bit Slice2 : hdlsllib/Logic and Bit Operations/Bit Slice  lidx=0  ridx=0
  Data Type Conversion2 : DataTypeConversion  OutDataTypeStr=boolean  RndMeth=Nearest  SaturateOnIntegerOverflow=off
  Switch2 : Switch  Criteria=u2 > Threshold  SaturateOnIntegerOverflow=off  InputSameDT=off
  out : Outport
  wires:
  in/1 -> Bit Shift2/1, Switch2/1, Bit Slice2/1
  Bit Shift2/1 -> Switch2/3
  Data Type Conversion2/1 -> Switch2/2
  Bit Slice2/1 -> Data Type Conversion2/1
  Switch2/1 -> out/1

== system UZ_EnDat_be4_adding_bidirectional_clk_shift/UZ_ENDAT/ManualDeserialize/padder/nibblepadding17/padding ==
  in : Inport
  Bit Shift2 : hdlsllib/Logic and Bit Operations/Bit Shift  mode=Shift Right Logical  N=1
  Bit Slice2 : hdlsllib/Logic and Bit Operations/Bit Slice  lidx=0  ridx=0
  Data Type Conversion2 : DataTypeConversion  OutDataTypeStr=boolean  RndMeth=Nearest  SaturateOnIntegerOverflow=off
  Switch2 : Switch  Criteria=u2 > Threshold  SaturateOnIntegerOverflow=off  InputSameDT=off
  out : Outport
  wires:
  in/1 -> Bit Shift2/1, Switch2/1, Bit Slice2/1
  Bit Shift2/1 -> Switch2/3
  Data Type Conversion2/1 -> Switch2/2
  Bit Slice2/1 -> Data Type Conversion2/1
  Switch2/1 -> out/1

== system UZ_EnDat_be4_adding_bidirectional_clk_shift/UZ_ENDAT/ManualDeserialize/padder/nibblepadding17/padding1 ==
  in : Inport
  Bit Shift2 : hdlsllib/Logic and Bit Operations/Bit Shift  mode=Shift Right Logical  N=1
  Bit Slice2 : hdlsllib/Logic and Bit Operations/Bit Slice  lidx=0  ridx=0
  Data Type Conversion2 : DataTypeConversion  OutDataTypeStr=boolean  RndMeth=Nearest  SaturateOnIntegerOverflow=off
  Switch2 : Switch  Criteria=u2 > Threshold  SaturateOnIntegerOverflow=off  InputSameDT=off
  out : Outport
  wires:
  in/1 -> Bit Shift2/1, Switch2/1, Bit Slice2/1
  Bit Shift2/1 -> Switch2/3
  Data Type Conversion2/1 -> Switch2/2
  Bit Slice2/1 -> Data Type Conversion2/1
  Switch2/1 -> out/1

== system UZ_EnDat_be4_adding_bidirectional_clk_shift/UZ_ENDAT/ManualDeserialize/padder/nibblepadding17/padding2 ==
  in : Inport
  Bit Shift2 : hdlsllib/Logic and Bit Operations/Bit Shift  mode=Shift Right Logical  N=1
  Bit Slice2 : hdlsllib/Logic and Bit Operations/Bit Slice  lidx=0  ridx=0
  Data Type Conversion2 : DataTypeConversion  OutDataTypeStr=boolean  RndMeth=Nearest  SaturateOnIntegerOverflow=off
  Switch2 : Switch  Criteria=u2 > Threshold  SaturateOnIntegerOverflow=off  InputSameDT=off
  out : Outport
  wires:
  in/1 -> Bit Shift2/1, Switch2/1, Bit Slice2/1
  Bit Shift2/1 -> Switch2/3
  Data Type Conversion2/1 -> Switch2/2
  Bit Slice2/1 -> Data Type Conversion2/1
  Switch2/1 -> out/1

== system UZ_EnDat_be4_adding_bidirectional_clk_shift/UZ_ENDAT/ManualDeserialize/padder/nibblepadding17/padding3 ==
  in : Inport
  Bit Shift2 : hdlsllib/Logic and Bit Operations/Bit Shift  mode=Shift Right Logical  N=1
  Bit Slice2 : hdlsllib/Logic and Bit Operations/Bit Slice  lidx=0  ridx=0
  Data Type Conversion2 : DataTypeConversion  OutDataTypeStr=boolean  RndMeth=Nearest  SaturateOnIntegerOverflow=off
  Switch2 : Switch  Criteria=u2 > Threshold  SaturateOnIntegerOverflow=off  InputSameDT=off
  out : Outport
  wires:
  in/1 -> Bit Shift2/1, Switch2/1, Bit Slice2/1
  Bit Shift2/1 -> Switch2/3
  Data Type Conversion2/1 -> Switch2/2
  Bit Slice2/1 -> Data Type Conversion2/1
  Switch2/1 -> out/1

== system UZ_EnDat_be4_adding_bidirectional_clk_shift/UZ_ENDAT/ManualDeserialize/padder/nibblepadding18/padding ==
  in : Inport
  Bit Shift2 : hdlsllib/Logic and Bit Operations/Bit Shift  mode=Shift Right Logical  N=1
  Bit Slice2 : hdlsllib/Logic and Bit Operations/Bit Slice  lidx=0  ridx=0
  Data Type Conversion2 : DataTypeConversion  OutDataTypeStr=boolean  RndMeth=Nearest  SaturateOnIntegerOverflow=off
  Switch2 : Switch  Criteria=u2 > Threshold  SaturateOnIntegerOverflow=off  InputSameDT=off
  out : Outport
  wires:
  in/1 -> Bit Shift2/1, Switch2/1, Bit Slice2/1
  Bit Shift2/1 -> Switch2/3
  Data Type Conversion2/1 -> Switch2/2
  Bit Slice2/1 -> Data Type Conversion2/1
  Switch2/1 -> out/1

== system UZ_EnDat_be4_adding_bidirectional_clk_shift/UZ_ENDAT/ManualDeserialize/padder/nibblepadding18/padding1 ==
  in : Inport
  Bit Shift2 : hdlsllib/Logic and Bit Operations/Bit Shift  mode=Shift Right Logical  N=1
  Bit Slice2 : hdlsllib/Logic and Bit Operations/Bit Slice  lidx=0  ridx=0
  Data Type Conversion2 : DataTypeConversion  OutDataTypeStr=boolean  RndMeth=Nearest  SaturateOnIntegerOverflow=off
  Switch2 : Switch  Criteria=u2 > Threshold  SaturateOnIntegerOverflow=off  InputSameDT=off
  out : Outport
  wires:
  in/1 -> Bit Shift2/1, Switch2/1, Bit Slice2/1
  Bit Shift2/1 -> Switch2/3
  Data Type Conversion2/1 -> Switch2/2
  Bit Slice2/1 -> Data Type Conversion2/1
  Switch2/1 -> out/1

== system UZ_EnDat_be4_adding_bidirectional_clk_shift/UZ_ENDAT/ManualDeserialize/padder/nibblepadding18/padding2 ==
  in : Inport
  Bit Shift2 : hdlsllib/Logic and Bit Operations/Bit Shift  mode=Shift Right Logical  N=1
  Bit Slice2 : hdlsllib/Logic and Bit Operations/Bit Slice  lidx=0  ridx=0
  Data Type Conversion2 : DataTypeConversion  OutDataTypeStr=boolean  RndMeth=Nearest  SaturateOnIntegerOverflow=off
  Switch2 : Switch  Criteria=u2 > Threshold  SaturateOnIntegerOverflow=off  InputSameDT=off
  out : Outport
  wires:
  in/1 -> Bit Shift2/1, Switch2/1, Bit Slice2/1
  Bit Shift2/1 -> Switch2/3
  Data Type Conversion2/1 -> Switch2/2
  Bit Slice2/1 -> Data Type Conversion2/1
  Switch2/1 -> out/1

== system UZ_EnDat_be4_adding_bidirectional_clk_shift/UZ_ENDAT/ManualDeserialize/padder/nibblepadding18/padding3 ==
  in : Inport
  Bit Shift2 : hdlsllib/Logic and Bit Operations/Bit Shift  mode=Shift Right Logical  N=1
  Bit Slice2 : hdlsllib/Logic and Bit Operations/Bit Slice  lidx=0  ridx=0
  Data Type Conversion2 : DataTypeConversion  OutDataTypeStr=boolean  RndMeth=Nearest  SaturateOnIntegerOverflow=off
  Switch2 : Switch  Criteria=u2 > Threshold  SaturateOnIntegerOverflow=off  InputSameDT=off
  out : Outport
  wires:
  in/1 -> Bit Shift2/1, Switch2/1, Bit Slice2/1
  Bit Shift2/1 -> Switch2/3
  Data Type Conversion2/1 -> Switch2/2
  Bit Slice2/1 -> Data Type Conversion2/1
  Switch2/1 -> out/1

== system UZ_EnDat_be4_adding_bidirectional_clk_shift/UZ_ENDAT/ManualDeserialize/padder/nibblepadding19/padding ==
  in : Inport
  Bit Shift2 : hdlsllib/Logic and Bit Operations/Bit Shift  mode=Shift Right Logical  N=1
  Bit Slice2 : hdlsllib/Logic and Bit Operations/Bit Slice  lidx=0  ridx=0
  Data Type Conversion2 : DataTypeConversion  OutDataTypeStr=boolean  RndMeth=Nearest  SaturateOnIntegerOverflow=off
  Switch2 : Switch  Criteria=u2 > Threshold  SaturateOnIntegerOverflow=off  InputSameDT=off
  out : Outport
  wires:
  in/1 -> Bit Shift2/1, Switch2/1, Bit Slice2/1
  Bit Shift2/1 -> Switch2/3
  Data Type Conversion2/1 -> Switch2/2
  Bit Slice2/1 -> Data Type Conversion2/1
  Switch2/1 -> out/1

== system UZ_EnDat_be4_adding_bidirectional_clk_shift/UZ_ENDAT/ManualDeserialize/padder/nibblepadding19/padding1 ==
  in : Inport
  Bit Shift2 : hdlsllib/Logic and Bit Operations/Bit Shift  mode=Shift Right Logical  N=1
  Bit Slice2 : hdlsllib/Logic and Bit Operations/Bit Slice  lidx=0  ridx=0
  Data Type Conversion2 : DataTypeConversion  OutDataTypeStr=boolean  RndMeth=Nearest  SaturateOnIntegerOverflow=off
  Switch2 : Switch  Criteria=u2 > Threshold  SaturateOnIntegerOverflow=off  InputSameDT=off
  out : Outport
  wires:
  in/1 -> Bit Shift2/1, Switch2/1, Bit Slice2/1
  Bit Shift2/1 -> Switch2/3
  Data Type Conversion2/1 -> Switch2/2
  Bit Slice2/1 -> Data Type Conversion2/1
  Switch2/1 -> out/1

== system UZ_EnDat_be4_adding_bidirectional_clk_shift/UZ_ENDAT/ManualDeserialize/padder/nibblepadding19/padding2 ==
  in : Inport
  Bit Shift2 : hdlsllib/Logic and Bit Operations/Bit Shift  mode=Shift Right Logical  N=1
  Bit Slice2 : hdlsllib/Logic and Bit Operations/Bit Slice  lidx=0  ridx=0
  Data Type Conversion2 : DataTypeConversion  OutDataTypeStr=boolean  RndMeth=Nearest  SaturateOnIntegerOverflow=off
  Switch2 : Switch  Criteria=u2 > Threshold  SaturateOnIntegerOverflow=off  InputSameDT=off
  out : Outport
  wires:
  in/1 -> Bit Shift2/1, Switch2/1, Bit Slice2/1
  Bit Shift2/1 -> Switch2/3
  Data Type Conversion2/1 -> Switch2/2
  Bit Slice2/1 -> Data Type Conversion2/1
  Switch2/1 -> out/1

== system UZ_EnDat_be4_adding_bidirectional_clk_shift/UZ_ENDAT/ManualDeserialize/padder/nibblepadding19/padding3 ==
  in : Inport
  Bit Shift2 : hdlsllib/Logic and Bit Operations/Bit Shift  mode=Shift Right Logical  N=1
  Bit Slice2 : hdlsllib/Logic and Bit Operations/Bit Slice  lidx=0  ridx=0
  Data Type Conversion2 : DataTypeConversion  OutDataTypeStr=boolean  RndMeth=Nearest  SaturateOnIntegerOverflow=off
  Switch2 : Switch  Criteria=u2 > Threshold  SaturateOnIntegerOverflow=off  InputSameDT=off
  out : Outport
  wires:
  in/1 -> Bit Shift2/1, Switch2/1, Bit Slice2/1
  Bit Shift2/1 -> Switch2/3
  Data Type Conversion2/1 -> Switch2/2
  Bit Slice2/1 -> Data Type Conversion2/1
  Switch2/1 -> out/1
